simulink model "newMasterTester"  (R2018b)
settings: Solver=FixedStepAuto  StartTime=0.0  StopTime=10.0  RelTol=1e-3
values from neighbouring files (symbols this model uses):
  BackUp_Role = 4    [HANcoder_E407_TTA_Group2_startup.m]
  Master_Role = 1    [HANcoder_E407_TTA_Group2_startup.m]    (also in HANcoder_E407_TTA_Template_startup.m)
  Slave_Role = 3    [HANcoder_E407_TTA_Group2_startup.m]    (also in HANcoder_E407_TTA_Template_startup.m = 2)
  Voter_Role = 2    [HANcoder_E407_TTA_Group2_startup.m]
libraries: simulink x3
settings Model: Creator=CheffryB  LastModifiedBy=cheff

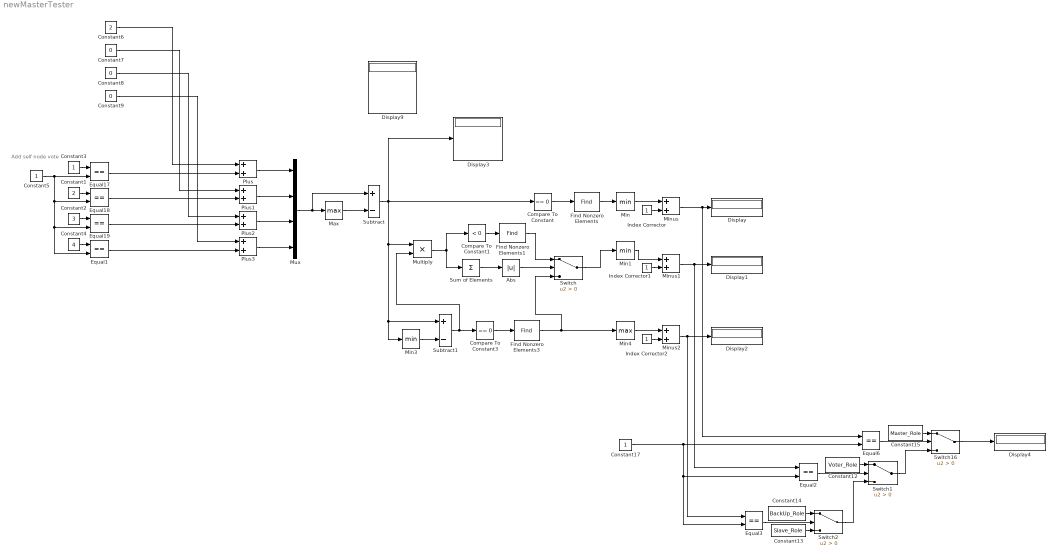
== system newMasterTester ==
  note: Add self node vote
  Abs : Abs
  Compare To Constant : simulink/Logic and Bit Operations/Compare To Constant  relop===  const=0  OutDataTypeStr=boolean
  Compare To Constant1 : simulink/Logic and Bit Operations/Compare To Constant  relop=<  const=0  OutDataTypeStr=boolean
  Compare To Constant3 : simulink/Logic and Bit Operations/Compare To Constant  relop===  const=0  OutDataTypeStr=boolean
  Constant1 : Constant  Value=2  OutDataTypeStr=single
  Constant12 : Constant  Value=Voter_Role
  Constant13 : Constant  Value=Slave_Role
  Constant14 : Constant  Value=BackUp_Role
  Constant15 : Constant  Value=Master_Role
  Constant17 : Constant  OutDataTypeStr=single
  Constant2 : Constant  Value=3  OutDataTypeStr=single
  Constant3 : Constant  OutDataTypeStr=single
  Constant4 : Constant  Value=4  OutDataTypeStr=single
  Constant5 : Constant  OutDataTypeStr=single
  Constant6 : Constant  Value=2  OutDataTypeStr=single
  Constant7 : Constant  Value=0  OutDataTypeStr=single
  Constant8 : Constant  Value=0  OutDataTypeStr=single
  Constant9 : Constant  Value=0  OutDataTypeStr=single
  Display{,1..4,9} (6 alike) : Display
  Equal{1..3,6,17..19} (7 alike) : RelationalOperator  Operator===  OutDataTypeStr=boolean  RndMeth=Simplest
  Find Nonzero Elements : Find  NumberOfInputDimensions=3  IndexMode=Zero-based  OutDataTypeStr=int32
  Find Nonzero Elements1 : Find  NumberOfInputDimensions=3  IndexMode=Zero-based  OutDataTypeStr=int32
  Find Nonzero Elements3 : Find  NumberOfInputDimensions=3  IndexMode=Zero-based  OutDataTypeStr=int32
  Index Corrector : Constant
  Index Corrector1 : Constant
  Index Corrector2 : Constant
  Max : MinMax  Function=max
  Min : MinMax
  Min1 : MinMax
  Min3 : MinMax
  Min4 : MinMax  Function=max
  Minus : Sum
  Minus1 : Sum
  Minus2 : Sum
  Multiply : Product
  Mux : Mux
  Plus{,1..3} (4 alike) : Sum
  Subtract : Sum  Inputs=+-
  Subtract1 : Sum  Inputs=+-
  Sum of Elements : Sum  Inputs=+
  Switch{,1..2,16} (4 alike) : Switch  Criteria=u2 > Threshold
  wires:
  Plus3/1 -> Mux/4
  Index Corrector1/1 -> Minus1/2
  Constant9/1 -> Plus3/1
  Compare To Constant/1 -> Find Nonzero Elements/1
  Plus2/1 -> Mux/3
  Mux/1 -> Subtract/1, Max/1
  Equal17/1 -> Plus/2
  Find Nonzero Elements/1 -> Min/1
  Constant3/1 -> Equal17/1
  Constant8/1 -> Plus2/1
  Min4/1 -> Minus2/1
  Constant5/1 -> Equal1/2, Equal19/2, Equal18/2, Equal17/2
  Plus/1 -> Mux/1
  Constant4/1 -> Equal1/1
  Equal18/1 -> Plus1/2
  Constant6/1 -> Plus/1
  Constant7/1 -> Plus1/1
  Index Corrector2/1 -> Minus2/2
  Index Corrector/1 -> Minus/2
  Equal1/1 -> Plus3/2
  Constant1/1 -> Equal18/1
  Equal19/1 -> Plus2/2
  Min/1 -> Minus/1
  Plus1/1 -> Mux/2
  Constant2/1 -> Equal19/1
  Equal2/1 -> Switch1/2
  Constant15/1 -> Switch16/1
  Equal6/1 -> Switch16/2
  Switch1/1 -> Switch16/3
  Switch16/1 -> Display4/1
  Constant12/1 -> Switch1/1
  Switch2/1 -> Switch1/3
  Minus1/1 -> Equal2/1, Display1/1
  Minus/1 -> Equal6/1, Display/1
  Constant13/1 -> Switch2/3
  Equal3/1 -> Switch2/2
  Constant14/1 -> Switch2/1
  Minus2/1 -> Equal3/1, Display2/1
  Constant17/1 -> Equal2/2, Equal3/2, Equal6/2
  Min3/1 -> Subtract1/2
  Subtract1/1 -> Compare To Constant3/1, Multiply/2
  Compare To Constant3/1 -> Find Nonzero Elements3/1
  Find Nonzero Elements3/1 -> Min4/1, Switch/3
  Subtract/1 -> Multiply/1, Subtract1/1, Min3/1, Compare To Constant/1, Display3/1
  Max/1 -> Subtract/2
  Compare To Constant1/1 -> Find Nonzero Elements1/1
  Multiply/1 -> Compare To Constant1/1, Sum of Elements/1
  Switch/1 -> Min1/1
  Min1/1 -> Minus1/1
  Sum of Elements/1 -> Abs/1
  Find Nonzero Elements1/1 -> Switch/1
  Abs/1 -> Switch/2
